simulink model "PX4_Run_Mode_R2017b"  (R2017b)
settings: Solver=FixedStepDiscrete  StartTime=0.0  StopTime=10.0  RelTol=1e-3  EnableMultiTasking=on
InitFcn:
  | run('InitFcn_R2017b_no_csc.m');
values from neighbouring files (symbols this model uses):
  A = Pixhawk_CSC.Parameter( {single([diag([1 1 1]) Ts*diag([1 1 1]); diag([0 0 0]) diag([1 1 1])]),'A'} )    [InitFcn.m]    (also in InitFcn_R2016b.m; InitFcn_R2017b_no_csc.m = single([diag([1 1 1]) Ts*diag([1 1 1]); diag([0 0 0]) diag([)
  app = Pixhawk_CSC.Parameter({single( [0.05; 0.05; 0.05]),'app'} )    [InitFcn.m]    (also in InitFcn_R2016b.m; InitFcn_R2017b_no_csc.m = single( [0.05; 0.05; 0.05]))
  B = Pixhawk_CSC.Parameter( {single([Ts^2/2*diag([1 1 1]); Ts*diag([1 1 1])]),'B'} )    [InitFcn.m]    (also in InitFcn_R2016b.m; InitFcn_R2017b_no_csc.m = single([Ts^2/2*diag([1 1 1]); Ts*diag([1 1 1])]))
  Beta = Pixhawk_CSC.Parameter({single( 0.02),'Beta'} )    [InitFcn.m]    (also in InitFcn_R2016b.m; InitFcn_R2017b_no_csc.m = single( 0.02))
  C = Pixhawk_CSC.Parameter( {single([diag([1 1 1]) 0*diag([1 1 1]); zeros(1,2) 1 zeros(1,3)]),'C'} )    [InitFcn.m]    (also in InitFcn_R2016b.m; InitFcn_R2017b_no_csc.m = single([diag([1 1 1]) 0*diag([1 1 1]); zeros(1,2) 1 zeros(1,)
  C1 = Pixhawk_CSC.Parameter({single( 1.08680),'C1'} )    [InitFcn.m]    (also in InitFcn_R2016b.m; InitFcn_R2017b_no_csc.m = single( 1.08680))
  C10 = Pixhawk_CSC.Parameter({single( 0.0000),'C10'} )    [InitFcn.m]    (also in InitFcn_R2016b.m; InitFcn_R2017b_no_csc.m = single( 0.0000))
  C11 = Pixhawk_CSC.Parameter({single(-0.2300),'C11'} )    [InitFcn.m]    (also in InitFcn_R2016b.m; InitFcn_R2017b_no_csc.m = single(-0.2300))
  C12 = Pixhawk_CSC.Parameter({single( 0.0000),'C12'} )    [InitFcn.m]    (also in InitFcn_R2016b.m; InitFcn_R2017b_no_csc.m = single( 0.0000))
  C13 = Pixhawk_CSC.Parameter({single( 0.8000),'C13'} )    [InitFcn.m]    (also in InitFcn_R2016b.m; InitFcn_R2017b_no_csc.m = single( 0.8000))
  C14 = Pixhawk_CSC.Parameter({single( 0.8000),'C14'} )    [InitFcn.m]    (also in InitFcn_R2016b.m; InitFcn_R2017b_no_csc.m = single( 0.8000))
  C15 = Pixhawk_CSC.Parameter({single( 1.73200),'C15'} )    [InitFcn.m]    (also in InitFcn_R2016b.m; InitFcn_R2017b_no_csc.m = single( 1.73200))
  C16 = Pixhawk_CSC.Parameter({single( 0.1000),'C16'} )    [InitFcn.m]    (also in InitFcn_R2016b.m; InitFcn_R2017b_no_csc.m = single( 0.1000))
  C17 = Pixhawk_CSC.Parameter({single( 0.1000),'C17'} )    [InitFcn.m]    (also in InitFcn_R2016b.m; InitFcn_R2017b_no_csc.m = single( 0.1000))
  C18 = Pixhawk_CSC.Parameter({single( 0.0500),'C18'} )    [InitFcn.m]    (also in InitFcn_R2016b.m; InitFcn_R2017b_no_csc.m = single( 0.0500))
  C19 = Pixhawk_CSC.Parameter({single( 0.6000),'C19'} )    [InitFcn.m]    (also in InitFcn_R2016b.m; InitFcn_R2017b_no_csc.m = single( 0.6000))
  C2 = Pixhawk_CSC.Parameter({single( 1.10468),'C2'} )    [InitFcn.m]    (also in InitFcn_R2016b.m; InitFcn_R2017b_no_csc.m = single( 1.10468))
  C20 = Pixhawk_CSC.Parameter({single( 0.6000),'C20'} )    [InitFcn.m]    (also in InitFcn_R2016b.m; InitFcn_R2017b_no_csc.m = single( 0.6000))
  C21 = Pixhawk_CSC.Parameter({single( 1.04558),'C21'} )    [InitFcn.m]    (also in InitFcn_R2016b.m; InitFcn_R2017b_no_csc.m = single( 1.04558))
  C22 = Pixhawk_CSC.Parameter({single( 0.0000),'C22'} )    [InitFcn.m]    (also in InitFcn_R2016b.m; InitFcn_R2017b_no_csc.m = single( 0.0000))
  C23 = Pixhawk_CSC.Parameter({single( 0.0000),'C23'} )    [InitFcn.m]    (also in InitFcn_R2016b.m; InitFcn_R2017b_no_csc.m = single( 0.0000))
  C24 = Pixhawk_CSC.Parameter({single(-11.0000),'C24'} )    [InitFcn.m]    (also in InitFcn_R2016b.m; InitFcn_R2017b_no_csc.m = single(-11.0000))
  C3 = Pixhawk_CSC.Parameter({single( 1.1980),'C3'} )    [InitFcn.m]    (also in InitFcn_R2016b.m; InitFcn_R2017b_no_csc.m = single( 1.1980))
  C4 = Pixhawk_CSC.Parameter({single( 0.0500),'C4'} )    [InitFcn.m]    (also in InitFcn_R2016b.m; InitFcn_R2017b_no_csc.m = single( 0.0500))
  C5 = Pixhawk_CSC.Parameter({single( 0.0500),'C5'} )    [InitFcn.m]    (also in InitFcn_R2016b.m; InitFcn_R2017b_no_csc.m = single( 0.0500))
  C6 = Pixhawk_CSC.Parameter({single( 0.0500),'C6'} )    [InitFcn.m]    (also in InitFcn_R2016b.m; InitFcn_R2017b_no_csc.m = single( 0.0500))
  C7 = Pixhawk_CSC.Parameter({single( 0.35937),'C7'} )    [InitFcn.m]    (also in InitFcn_R2016b.m; InitFcn_R2017b_no_csc.m = single( 0.35937))
  C8 = Pixhawk_CSC.Parameter({single( 0.36528),'C8'} )    [InitFcn.m]    (also in InitFcn_R2016b.m; InitFcn_R2017b_no_csc.m = single( 0.36528))
  C9 = Pixhawk_CSC.Parameter({single( 0.53311),'C9'} )    [InitFcn.m]    (also in InitFcn_R2016b.m; InitFcn_R2017b_no_csc.m = single( 0.53311))
  C_1 = Pixhawk_CSC.Parameter( {single([diag([1 1 1]) 0*diag([1 1 1])]),'C1'} )    [InitFcn.m]    (also in InitFcn_R2016b.m; InitFcn_R2017b_no_csc.m = single([diag([1 1 1]) 0*diag([1 1 1])]))
  CAL_ACC0_XOFFSET = Pixhawk_CSC.Parameter( {single( 0.122052  ),'CAL_ACC0_XOFFSET'} )    [InitFcn.m]    (also in InitFcn_R2016b.m; InitFcn_R2017b_no_csc.m = single( 0.122052  ))
  CAL_ACC0_XXSCALE = Pixhawk_CSC.Parameter( {single(  1.01218    ),'CAL_ACC0_XXSCALE'} )    [InitFcn.m]    (also in InitFcn_R2016b.m; InitFcn_R2017b_no_csc.m = single(  1.01218    ))
  CAL_ACC0_XYSCALE = Pixhawk_CSC.Parameter( {single( -0.00443301 ),'CAL_ACC0_XYSCALE'} )    [InitFcn.m]    (also in InitFcn_R2016b.m; InitFcn_R2017b_no_csc.m = single( -0.00443301 ))
  CAL_ACC0_XZSCALE = Pixhawk_CSC.Parameter( {single( -0.00505793 ),'CAL_ACC0_XZSCALE'} )    [InitFcn.m]    (also in InitFcn_R2016b.m; InitFcn_R2017b_no_csc.m = single( -0.00505793 ))
  CAL_ACC0_YOFFSET = Pixhawk_CSC.Parameter( {single( 0.00281205),'CAL_ACC0_YOFFSET'} )    [InitFcn.m]    (also in InitFcn_R2016b.m; InitFcn_R2017b_no_csc.m = single( 0.00281205))
  CAL_ACC0_YXSCALE = Pixhawk_CSC.Parameter( {single( -0.00443301 ),'CAL_ACC0_YXSCALE'} )    [InitFcn.m]    (also in InitFcn_R2016b.m; InitFcn_R2017b_no_csc.m = single( -0.00443301 ))
  CAL_ACC0_YYSCALE = Pixhawk_CSC.Parameter( {single(  1.00234    ),'CAL_ACC0_YYSCALE'} )    [InitFcn.m]    (also in InitFcn_R2016b.m; InitFcn_R2017b_no_csc.m = single(  1.00234    ))
  CAL_ACC0_YZSCALE = Pixhawk_CSC.Parameter( {single(  0.0160883  ),'CAL_ACC0_YZSCALE'} )    [InitFcn.m]    (also in InitFcn_R2016b.m; InitFcn_R2017b_no_csc.m = single(  0.0160883  ))
  CAL_ACC0_ZOFFSET = Pixhawk_CSC.Parameter( {single(-0.0298121 ),'CAL_ACC0_ZOFFSET'} )    [InitFcn.m]    (also in InitFcn_R2016b.m; InitFcn_R2017b_no_csc.m = single(-0.0298121 ))
  CAL_ACC0_ZXSCALE = Pixhawk_CSC.Parameter( {single( -0.00505793 ),'CAL_ACC0_ZXSCALE'} )    [InitFcn.m]    (also in InitFcn_R2016b.m; InitFcn_R2017b_no_csc.m = single( -0.00505793 ))
  CAL_ACC0_ZYSCALE = Pixhawk_CSC.Parameter( {single(  0.0160883  ),'CAL_ACC0_ZYSCALE'} )    [InitFcn.m]    (also in InitFcn_R2016b.m; InitFcn_R2017b_no_csc.m = single(  0.0160883  ))
  CAL_ACC0_ZZSCALE = Pixhawk_CSC.Parameter( {single(  0.983604   ),'CAL_ACC0_ZZSCALE'} )    [InitFcn.m]    (also in InitFcn_R2016b.m; InitFcn_R2017b_no_csc.m = single(  0.983604   ))
  CAL_BAR_OFFSET = Pixhawk_CSC.Parameter( {single( -20.8468),'CAL_BAR_OFFSET'} )    [InitFcn.m]    (also in InitFcn_R2016b.m; InitFcn_R2017b_no_csc.m = single( -20.8468))
  CAL_BAR_SCALE = Pixhawk_CSC.Parameter( {single(   1.0632),'CAL_BAR_SCALE'} )    [InitFcn.m]    (also in InitFcn_R2016b.m; InitFcn_R2017b_no_csc.m = single(   1.0632))
  CAL_BAT0_XOFFSET = Pixhawk_CSC.Parameter( {single( 0.0000),'CAL_BAT0_XOFFSET'} )    [InitFcn.m]    (also in InitFcn_R2016b.m; InitFcn_R2017b_no_csc.m = single( 0.0000))
  CAL_BAT0_XXSCALE = Pixhawk_CSC.Parameter( {single(  1.0000),'CAL_BAT0_XXSCALE'} )    [InitFcn.m]    (also in InitFcn_R2016b.m; InitFcn_R2017b_no_csc.m = single(  1.0000))
  CAL_BAT0_XYSCALE = Pixhawk_CSC.Parameter( {single(  0.0000),'CAL_BAT0_XYSCALE'} )    [InitFcn.m]    (also in InitFcn_R2016b.m; InitFcn_R2017b_no_csc.m = single(  0.0000))
  CAL_BAT0_XZSCALE = Pixhawk_CSC.Parameter( {single(  0.0000),'CAL_BAT0_XZSCALE'} )    [InitFcn.m]    (also in InitFcn_R2016b.m; InitFcn_R2017b_no_csc.m = single(  0.0000))
  CAL_BAT0_YOFFSET = Pixhawk_CSC.Parameter( {single( 0.0000),'CAL_BAT0_YOFFSET'} )    [InitFcn.m]    (also in InitFcn_R2016b.m; InitFcn_R2017b_no_csc.m = single( 0.0000))
  CAL_BAT0_YXSCALE = Pixhawk_CSC.Parameter( {single(  0.0000),'CAL_BAT0_YXSCALE'} )    [InitFcn.m]    (also in InitFcn_R2016b.m; InitFcn_R2017b_no_csc.m = single(  0.0000))
  CAL_BAT0_YYSCALE = Pixhawk_CSC.Parameter( {single(  1.0000),'CAL_BAT0_YYSCALE'} )    [InitFcn.m]    (also in InitFcn_R2016b.m; InitFcn_R2017b_no_csc.m = single(  1.0000))
  CAL_BAT0_YZSCALE = Pixhawk_CSC.Parameter( {single(  0.0000),'CAL_BAT0_YZSCALE'} )    [InitFcn.m]    (also in InitFcn_R2016b.m; InitFcn_R2017b_no_csc.m = single(  0.0000))
  CAL_BAT0_ZOFFSET = Pixhawk_CSC.Parameter( {single( 0.0000),'CAL_BAT0_ZOFFSET'} )    [InitFcn.m]    (also in InitFcn_R2016b.m; InitFcn_R2017b_no_csc.m = single( 0.0000))
  CAL_BAT0_ZXSCALE = Pixhawk_CSC.Parameter( {single(  0.0000),'CAL_BAT0_ZXSCALE'} )    [InitFcn.m]    (also in InitFcn_R2016b.m; InitFcn_R2017b_no_csc.m = single(  0.0000))
  CAL_BAT0_ZYSCALE = Pixhawk_CSC.Parameter( {single(  0.0000),'CAL_BAT0_ZYSCALE'} )    [InitFcn.m]    (also in InitFcn_R2016b.m; InitFcn_R2017b_no_csc.m = single(  0.0000))
  CAL_BAT0_ZZSCALE = Pixhawk_CSC.Parameter( {single(  1.0000),'CAL_BAT0_ZZSCALE'} )    [InitFcn.m]    (also in InitFcn_R2016b.m; InitFcn_R2017b_no_csc.m = single(  1.0000))
  CAL_GPS0_XOFFSET = Pixhawk_CSC.Parameter( {single( 0.0000),'CAL_GPS0_XOFFSET'} )    [InitFcn.m]    (also in InitFcn_R2016b.m; InitFcn_R2017b_no_csc.m = single( 0.0000))
  CAL_GPS0_XXSCALE = Pixhawk_CSC.Parameter( {single(  0.0100),'CAL_GPS0_XXSCALE'} )    [InitFcn.m]    (also in InitFcn_R2016b.m; InitFcn_R2017b_no_csc.m = single(  0.0100))
  CAL_GPS0_XYSCALE = Pixhawk_CSC.Parameter( {single(  0.0000),'CAL_GPS0_XYSCALE'} )    [InitFcn.m]    (also in InitFcn_R2016b.m; InitFcn_R2017b_no_csc.m = single(  0.0000))
  CAL_GPS0_XZSCALE = Pixhawk_CSC.Parameter( {single(  0.0000),'CAL_GPS0_XZSCALE'} )    [InitFcn.m]    (also in InitFcn_R2016b.m; InitFcn_R2017b_no_csc.m = single(  0.0000))
  CAL_GPS0_YOFFSET = Pixhawk_CSC.Parameter( {single( 0.0000),'CAL_GPS0_YOFFSET'} )    [InitFcn.m]    (also in InitFcn_R2016b.m; InitFcn_R2017b_no_csc.m = single( 0.0000))
  CAL_GPS0_YXSCALE = Pixhawk_CSC.Parameter( {single(  0.0000),'CAL_GPS0_YXSCALE'} )    [InitFcn.m]    (also in InitFcn_R2016b.m; InitFcn_R2017b_no_csc.m = single(  0.0000))
  CAL_GPS0_YYSCALE = Pixhawk_CSC.Parameter( {single(  0.0100),'CAL_GPS0_YYSCALE'} )    [InitFcn.m]    (also in InitFcn_R2016b.m; InitFcn_R2017b_no_csc.m = single(  0.0100))
  CAL_GPS0_YZSCALE = Pixhawk_CSC.Parameter( {single(  0.0000),'CAL_GPS0_YZSCALE'} )    [InitFcn.m]    (also in InitFcn_R2016b.m; InitFcn_R2017b_no_csc.m = single(  0.0000))
  CAL_GPS0_ZOFFSET = Pixhawk_CSC.Parameter( {single( 0.0000),'CAL_GPS0_ZOFFSET'} )    [InitFcn.m]    (also in InitFcn_R2016b.m; InitFcn_R2017b_no_csc.m = single( 0.0000))
  CAL_GPS0_ZXSCALE = Pixhawk_CSC.Parameter( {single(  0.0000),'CAL_GPS0_ZXSCALE'} )    [InitFcn.m]    (also in InitFcn_R2016b.m; InitFcn_R2017b_no_csc.m = single(  0.0000))
  CAL_GPS0_ZYSCALE = Pixhawk_CSC.Parameter( {single(  0.0000),'CAL_GPS0_ZYSCALE'} )    [InitFcn.m]    (also in InitFcn_R2016b.m; InitFcn_R2017b_no_csc.m = single(  0.0000))
  CAL_GPS0_ZZSCALE = Pixhawk_CSC.Parameter( {single( -0.0010),'CAL_GPS0_ZZSCALE'} )    [InitFcn.m]    (also in InitFcn_R2016b.m; InitFcn_R2017b_no_csc.m = single( -0.0010))
  CAL_GYRO0_XXSCALE = Pixhawk_CSC.Parameter( {single(0.992736),'CAL_GYRO0_XXSCALE'} )    [InitFcn.m]    (also in InitFcn_R2016b.m; InitFcn_R2017b_no_csc.m = single(0.992736))
  CAL_GYRO0_XYSCALE = Pixhawk_CSC.Parameter( {single(0.0000),'CAL_GYRO0_XYSCALE'} )    [InitFcn.m]    (also in InitFcn_R2016b.m; InitFcn_R2017b_no_csc.m = single(0.0000))
  CAL_GYRO0_XZSCALE = Pixhawk_CSC.Parameter( {single(0.0000),'CAL_GYRO0_XZSCALE'} )    [InitFcn.m]    (also in InitFcn_R2016b.m; InitFcn_R2017b_no_csc.m = single(0.0000))
  CAL_GYRO0_YXSCALE = Pixhawk_CSC.Parameter( {single(0.0000),'CAL_GYRO0_YXSCALE'} )    [InitFcn.m]    (also in InitFcn_R2016b.m; InitFcn_R2017b_no_csc.m = single(0.0000))
  CAL_GYRO0_YYSCALE = Pixhawk_CSC.Parameter( {single(1.01609),'CAL_GYRO0_YYSCALE'} )    [InitFcn.m]    (also in InitFcn_R2016b.m; InitFcn_R2017b_no_csc.m = single(1.01609))
  CAL_GYRO0_YZSCALE = Pixhawk_CSC.Parameter( {single(0.0000),'CAL_GYRO0_YZSCALE'} )    [InitFcn.m]    (also in InitFcn_R2016b.m; InitFcn_R2017b_no_csc.m = single(0.0000))
  CAL_GYRO0_ZXSCALE = Pixhawk_CSC.Parameter( {single(0.0000),'CAL_GYRO0_ZXSCALE'} )    [InitFcn.m]    (also in InitFcn_R2016b.m; InitFcn_R2017b_no_csc.m = single(0.0000))
  CAL_GYRO0_ZYSCALE = Pixhawk_CSC.Parameter( {single(0.0000),'CAL_GYRO0_ZYSCALE'} )    [InitFcn.m]    (also in InitFcn_R2016b.m; InitFcn_R2017b_no_csc.m = single(0.0000))
  CAL_GYRO0_ZZSCALE = Pixhawk_CSC.Parameter( {single(1.03003),'CAL_GYRO0_ZZSCALE'} )    [InitFcn.m]    (also in InitFcn_R2016b.m; InitFcn_R2017b_no_csc.m = single(1.03003))
  CAL_MAG0_XCURCOR = Pixhawk_CSC.Parameter( {single( 0.0017     ),'CAL_MAG0_XCURCOR'} )    [InitFcn.m]    (also in InitFcn_R2016b.m; InitFcn_R2017b_no_csc.m = single( 0.0017     ))
  CAL_MAG0_XOFFSET = Pixhawk_CSC.Parameter( {single( 0.0446372  ),'CAL_MAG0_XOFFSET'} )    [InitFcn.m]    (also in InitFcn_R2016b.m; InitFcn_R2017b_no_csc.m = single( 0.0446372  ))
  CAL_MAG0_XXSCALE = Pixhawk_CSC.Parameter( {single(  1.01563   ),'CAL_MAG0_XXSCALE'} )    [InitFcn.m]    (also in InitFcn_R2016b.m; InitFcn_R2017b_no_csc.m = single(  1.01563   ))
  CAL_MAG0_XYSCALE = Pixhawk_CSC.Parameter( {single( -0.0612061 ),'CAL_MAG0_XYSCALE'} )    [InitFcn.m]    (also in InitFcn_R2016b.m; InitFcn_R2017b_no_csc.m = single( -0.0612061 ))
  CAL_MAG0_XZSCALE = Pixhawk_CSC.Parameter( {single( -0.011532  ),'CAL_MAG0_XZSCALE'} )    [InitFcn.m]    (also in InitFcn_R2016b.m; InitFcn_R2017b_no_csc.m = single( -0.011532  ))
  CAL_MAG0_YCURCOR = Pixhawk_CSC.Parameter( {single(-0.0075     ),'CAL_MAG0_YCURCOR'} )    [InitFcn.m]    (also in InitFcn_R2016b.m; InitFcn_R2017b_no_csc.m = single(-0.0075     ))
  CAL_MAG0_YOFFSET = Pixhawk_CSC.Parameter( {single( 0.0700776  ),'CAL_MAG0_YOFFSET'} )    [InitFcn.m]    (also in InitFcn_R2016b.m; InitFcn_R2017b_no_csc.m = single( 0.0700776  ))
  CAL_MAG0_YXSCALE = Pixhawk_CSC.Parameter( {single( -0.0612061 ),'CAL_MAG0_YXSCALE'} )    [InitFcn.m]    (also in InitFcn_R2016b.m; InitFcn_R2017b_no_csc.m = single( -0.0612061 ))
  CAL_MAG0_YYSCALE = Pixhawk_CSC.Parameter( {single(  1.00593   ),'CAL_MAG0_YYSCALE'} )    [InitFcn.m]    (also in InitFcn_R2016b.m; InitFcn_R2017b_no_csc.m = single(  1.00593   ))
  CAL_MAG0_YZSCALE = Pixhawk_CSC.Parameter( {single(  0.0144582 ),'CAL_MAG0_YZSCALE'} )    [InitFcn.m]    (also in InitFcn_R2016b.m; InitFcn_R2017b_no_csc.m = single(  0.0144582 ))
  CAL_MAG0_ZCURCOR = Pixhawk_CSC.Parameter( {single(-0.0080     ),'CAL_MAG0_ZCURCOR'} )    [InitFcn.m]    (also in InitFcn_R2016b.m; InitFcn_R2017b_no_csc.m = single(-0.0080     ))
  CAL_MAG0_ZOFFSET = Pixhawk_CSC.Parameter( {single( 0.00201742 ),'CAL_MAG0_ZOFFSET'} )    [InitFcn.m]    (also in InitFcn_R2016b.m; InitFcn_R2017b_no_csc.m = single( 0.00201742 ))
  CAL_MAG0_ZXSCALE = Pixhawk_CSC.Parameter( {single( -0.011532  ),'CAL_MAG0_ZXSCALE'} )    [InitFcn.m]    (also in InitFcn_R2016b.m; InitFcn_R2017b_no_csc.m = single( -0.011532  ))
  CAL_MAG0_ZYSCALE = Pixhawk_CSC.Parameter( {single(  0.0144582 ),'CAL_MAG0_ZYSCALE'} )    [InitFcn.m]    (also in InitFcn_R2016b.m; InitFcn_R2017b_no_csc.m = single(  0.0144582 ))
  CAL_MAG0_ZZSCALE = Pixhawk_CSC.Parameter( {single(  0.986813  ),'CAL_MAG0_ZZSCALE'} )    [InitFcn.m]    (also in InitFcn_R2016b.m; InitFcn_R2017b_no_csc.m = single(  0.986813  ))
  CAL_SONAR_OFFSET = Pixhawk_CSC.Parameter( {single( -6.8730),'CAL_SONAR_OFFSET'} )    [InitFcn.m]    (also in InitFcn_R2016b.m; InitFcn_R2017b_no_csc.m = single( -6.8730))
  CAL_SONAR_SCALE = Pixhawk_CSC.Parameter( {single(-438.1875),'CAL_SONAR_SCALE'} )    [InitFcn.m]    (also in InitFcn_R2016b.m; InitFcn_R2017b_no_csc.m = single(-438.1875))
  COM_RATE = double(10)    [InitFcn.m]    (also in InitFcn_R2016b.m; InitFcn_R2017b_no_csc.m)
  D = Pixhawk_CSC.Parameter( {single(zeros(size(C.Value,1), size(B.Value,2))),'D'} )    [InitFcn.m]    (also in InitFcn_R2016b.m; InitFcn_R2017b_no_csc.m = single(zeros(size(C,1), size(B,2))))
  Dip0 = Pixhawk_CSC.Parameter({single( 1.2),'Dip0'} )    [InitFcn.m]    (also in InitFcn_R2016b.m; InitFcn_R2017b_no_csc.m = single( 1.2))
  I = Pixhawk_CSC.Parameter( {single(eye(size(Q.Value))),'I'} )    [InitFcn.m]    (also in InitFcn_R2016b.m; InitFcn_R2017b_no_csc.m = single(eye(size(Q))))
  Jxx = Pixhawk_CSC.Parameter( {single(J(1,1)),'Jxx'} )    [InitFcn.m]    (also in InitFcn_R2016b.m; InitFcn_R2017b_no_csc.m = single(J(1,1)))
  Jyy = Pixhawk_CSC.Parameter( {single(J(2,2)),'Jyy'} )    [InitFcn.m]    (also in InitFcn_R2016b.m; InitFcn_R2017b_no_csc.m = single(J(2,2)))
  Jzz = Pixhawk_CSC.Parameter( {single(J(3,3)),'Jzz'} )    [InitFcn.m]    (also in InitFcn_R2016b.m; InitFcn_R2017b_no_csc.m = single(J(3,3)))
  Kapp = Pixhawk_CSC.Parameter({single( 1.2),'Kapp'} )    [InitFcn.m]    (also in InitFcn_R2016b.m; InitFcn_R2017b_no_csc.m = single( 1.2))
  Kx = Pixhawk_CSC.Parameter({single( Kx),'Kx'} )    [InitFcn.m]    (also in InitFcn_R2016b.m = Pixhawk_CSC.Parameter({single( [0.60 0.9]),'Kx'} ); InitFcn_R2017b_no_csc.m = single( [0.60 0.9]))
  Ky = Pixhawk_CSC.Parameter({single( Ky),'Ky'} )    [InitFcn.m]    (also in InitFcn_R2016b.m = Pixhawk_CSC.Parameter({single( [0.4 0.9]),'Ky'} ); InitFcn_R2017b_no_csc.m = single( [0.4 0.9]))
  LPF_REF_DEN = Pixhawk_CSC.Parameter( {single([1.0000 -0.8187]),'LPF_REF_DEN'} )    [InitFcn.m]    (also in InitFcn_R2016b.m; InitFcn_R2017b_no_csc.m = single([1.0000 -0.8187]))
  LPF_REF_NUM = Pixhawk_CSC.Parameter( {single([0.0000  0.1813]),'LPF_REF_NUM'} )    [InitFcn.m]    (also in InitFcn_R2016b.m; InitFcn_R2017b_no_csc.m = single([0.0000  0.1813]))
  m0 = Pixhawk_CSC.Parameter({single( 0.452857),'m0'} )    [InitFcn.m]    (also in InitFcn_R2016b.m; InitFcn_R2017b_no_csc.m = single( 0.452857))
  mn = [0.01; 0.01; 0.01; 0.01]    [InitFcn.m]    (also in InitFcn_R2016b.m; InitFcn_R2017b_no_csc.m)
  MOV_AVG_WINDOW = Pixhawk_CSC.Parameter( {single(100),'MOV_AVG_WINDOW'} )    [InitFcn.m]    (also in InitFcn_R2016b.m; InitFcn_R2017b_no_csc.m = single(100))
  Ox0 = Pixhawk_CSC.Parameter({single(O_x0),'Ox0'} )    [InitFcn.m]    (also in InitFcn_R2016b.m; InitFcn_R2017b_no_csc.m = single(O_x0))
  Oxa = Pixhawk_CSC.Parameter({single(O_x.a),'Oxa'} )    [InitFcn.m]    (also in InitFcn_R2016b.m; InitFcn_R2017b_no_csc.m = single(O_x.a))
  Oxb = Pixhawk_CSC.Parameter({single(O_x.b),'Oxb'} )    [InitFcn.m]    (also in InitFcn_R2016b.m; InitFcn_R2017b_no_csc.m = single(O_x.b))
  Oxc = Pixhawk_CSC.Parameter({single(O_x.c),'Oxc'} )    [InitFcn.m]    (also in InitFcn_R2016b.m; InitFcn_R2017b_no_csc.m = single(O_x.c))
  Oxd = Pixhawk_CSC.Parameter({single(O_x.d),'Oxd'} )    [InitFcn.m]    (also in InitFcn_R2016b.m; InitFcn_R2017b_no_csc.m = single(O_x.d))
  Oy0 = Pixhawk_CSC.Parameter({single(O_y0),'Oy0'} )    [InitFcn.m]    (also in InitFcn_R2016b.m; InitFcn_R2017b_no_csc.m = single(O_y0))
  Oya = Pixhawk_CSC.Parameter({single(O_y.a),'Oya'} )    [InitFcn.m]    (also in InitFcn_R2016b.m; InitFcn_R2017b_no_csc.m = single(O_y.a))
  Oyb = Pixhawk_CSC.Parameter({single(O_y.b),'Oyb'} )    [InitFcn.m]    (also in InitFcn_R2016b.m; InitFcn_R2017b_no_csc.m = single(O_y.b))
  Oyc = Pixhawk_CSC.Parameter({single(O_y.c),'Oyc'} )    [InitFcn.m]    (also in InitFcn_R2016b.m; InitFcn_R2017b_no_csc.m = single(O_y.c))
  Oyd = Pixhawk_CSC.Parameter({single(O_y.d),'Oyd'} )    [InitFcn.m]    (also in InitFcn_R2016b.m; InitFcn_R2017b_no_csc.m = single(O_y.d))
  Oz0 = Pixhawk_CSC.Parameter({single(O_z0),'Oz0'} )    [InitFcn.m]    (also in InitFcn_R2016b.m; InitFcn_R2017b_no_csc.m = single(O_z0))
  ... (+53 more)
undefined symbols (not defined in the file or in its folder): AccX, AccY, AccZ, Altitude, ax, ay, az, Current, FILTER_N, GPS_TS, GyroX, GyroY, GyroZ, Latitude, Longitude, M1_PWM, M2_PWM, M3_PWM, M4_PWM, MagX, MagY, MagZ, mAH, MOTOR, phi, Position_TS, psi, PX4_TUNE_ENUM, RGBLED_COLOR_ENUM, RGBLED_MODE_ENUM, S_AccX, S_AccY, S_AccZ, S_Altitude, S_Baro, S_Current, S_GyroX, S_GyroY, S_GyroZ, S_Latitude, S_Longitude, S_MagX, S_MagY, S_MagZ, S_mAH, S_N_Sat, S_Voltage, T_PITCH, T_ROLL, T_THROTTLE, theta, v, Voltage, w, wx, wxd, wy, wyd, wz ... (+4)
libraries: simulink x31, pixhawk_slib_sensors_actuators x7, pixhawk_slib_ADC_serial x5, pixhawk_slib_misc_utils x3, etargetslib x2
(part 6 of 7)

== system PX4_Run_Mode_R2017b/SENSOR_FILTER/Fixed Bias removal and scaling/Parameter Bus Creation/Kalman Filter/C matrix ==
  C matrix In : Inport
  Bus Creator : BusCreator  Inputs=24
  Data Type Conversion : DataTypeConversion  OutDataTypeStr=single
  Demux : Demux  Outputs=24
  C matrix Out : Outport
  wires:
  C matrix In/1 -> Data Type Conversion/1
  Bus Creator/1 -> C matrix Out/1  "C matrix"
  Demux/8 -> Bus Creator/8  "C42"
  Demux/10 -> Bus Creator/10  "C23"
  Demux/5 -> Bus Creator/5  "C12"
  Demux/13 -> Bus Creator/13  "C14"
  Demux/9 -> Bus Creator/9  "C13"
  Demux/18 -> Bus Creator/18  "C25"
  Demux/6 -> Bus Creator/6  "C22"
  Demux/12 -> Bus Creator/12  "C43"
  Demux/4 -> Bus Creator/4  "C41"
  Demux/7 -> Bus Creator/7  "C32"
  Demux/17 -> Bus Creator/17  "C15"
  Demux/11 -> Bus Creator/11  "C33"
  Demux/15 -> Bus Creator/15  "C34"
  Demux/3 -> Bus Creator/3  "C31"
  Demux/14 -> Bus Creator/14  "C24"
  Demux/16 -> Bus Creator/16  "C44"
  Demux/2 -> Bus Creator/2  "C21"
  Demux/1 -> Bus Creator/1  "C11"
  Data Type Conversion/1 -> Demux/1
  Demux/22 -> Bus Creator/22  "C26"
  Demux/23 -> Bus Creator/23  "C36"
  Demux/20 -> Bus Creator/20  "C45"
  Demux/19 -> Bus Creator/19  "C35"
  Demux/21 -> Bus Creator/21  "C16"
  Demux/24 -> Bus Creator/24  "C46"

== system PX4_Run_Mode_R2017b/SENSOR_FILTER/Fixed Bias removal and scaling/Parameter Bus Creation/Kalman Filter/D matrix ==
  D matrix In : Inport
  Bus Creator : BusCreator  Inputs=12
  Data Type Conversion : DataTypeConversion  OutDataTypeStr=single
  Demux : Demux  Outputs=12
  D matrix Out : Outport
  wires:
  D matrix In/1 -> Data Type Conversion/1
  Bus Creator/1 -> D matrix Out/1  "D matrix"
  Demux/8 -> Bus Creator/8  "D42"
  Demux/5 -> Bus Creator/5  "D12"
  Demux/9 -> Bus Creator/9  "D13"
  Demux/6 -> Bus Creator/6  "D22"
  Demux/4 -> Bus Creator/4  "D41"
  Demux/7 -> Bus Creator/7  "D32"
  Demux/3 -> Bus Creator/3  "D31"
  Demux/2 -> Bus Creator/2  "D21"
  Demux/1 -> Bus Creator/1  "D11"
  Data Type Conversion/1 -> Demux/1
  Demux/10 -> Bus Creator/10  "D23"
  Demux/11 -> Bus Creator/11  "D33"
  Demux/12 -> Bus Creator/12  "D43"

== system PX4_Run_Mode_R2017b/SENSOR_FILTER/Fixed Bias removal and scaling/Parameter Bus Creation/Kalman Filter/Q matrix ==
  Q matrix In : Inport
  Bus Creator : BusCreator  Inputs=36
  Data Type Conversion : DataTypeConversion  OutDataTypeStr=single
  Demux : Demux  Outputs=36
  Q matrix Out : Outport
  wires:
  Q matrix In/1 -> Data Type Conversion/1
  Bus Creator/1 -> Q matrix Out/1  "Q matrix"
  Demux/8 -> Bus Creator/8  "Q22"
  Demux/10 -> Bus Creator/10  "Q42"
  Demux/19 -> Bus Creator/19  "Q14"
  Demux/5 -> Bus Creator/5  "Q51"
  Demux/13 -> Bus Creator/13  "Q13"
  Demux/20 -> Bus Creator/20  "Q24"
  Demux/9 -> Bus Creator/9  "Q32"
  Demux/18 -> Bus Creator/18  "Q63"
  Demux/6 -> Bus Creator/6  "Q61"
  Demux/12 -> Bus Creator/12  "Q62"
  Demux/4 -> Bus Creator/4  "Q41"
  Demux/7 -> Bus Creator/7  "Q12"
  Demux/17 -> Bus Creator/17  "Q53"
  Demux/11 -> Bus Creator/11  "Q52"
  Demux/15 -> Bus Creator/15  "Q33"
  Demux/3 -> Bus Creator/3  "Q31"
  Demux/21 -> Bus Creator/21  "Q34"
  Demux/14 -> Bus Creator/14  "Q23"
  Demux/16 -> Bus Creator/16  "Q43"
  Demux/34 -> Bus Creator/34  "Q46"
  Demux/28 -> Bus Creator/28  "Q45"
  Demux/30 -> Bus Creator/30  "Q65"
  Demux/27 -> Bus Creator/27  "Q35"
  Demux/29 -> Bus Creator/29  "Q55"
  Demux/31 -> Bus Creator/31  "Q16"
  Demux/32 -> Bus Creator/32  "Q26"
  Demux/22 -> Bus Creator/22  "Q44"
  Demux/24 -> Bus Creator/24  "Q64"
  Demux/33 -> Bus Creator/33  "Q36"
  Demux/23 -> Bus Creator/23  "Q54"
  Demux/36 -> Bus Creator/36  "Q66"
  Demux/25 -> Bus Creator/25  "Q15"
  Demux/26 -> Bus Creator/26  "Q25"
  Demux/35 -> Bus Creator/35  "Q56"
  Demux/2 -> Bus Creator/2  "Q21"
  Demux/1 -> Bus Creator/1  "Q11"
  Data Type Conversion/1 -> Demux/1

== system PX4_Run_Mode_R2017b/SENSOR_FILTER/Fixed Bias removal and scaling/Parameter Bus Creation/Kalman Filter/R matrix ==
  R matrix In : Inport
  Bus Creator : BusCreator  Inputs=16
  Data Type Conversion : DataTypeConversion  OutDataTypeStr=single
  Demux : Demux  Outputs=16
  R matrix Out : Outport
  wires:
  R matrix In/1 -> Data Type Conversion/1
  Bus Creator/1 -> R matrix Out/1  "R matrix"
  Demux/8 -> Bus Creator/8  "R42"
  Demux/5 -> Bus Creator/5  "R12"
  Demux/9 -> Bus Creator/9  "R13"
  Demux/6 -> Bus Creator/6  "R22"
  Demux/4 -> Bus Creator/4  "R41"
  Demux/7 -> Bus Creator/7  "R32"
  Demux/3 -> Bus Creator/3  "R31"
  Demux/2 -> Bus Creator/2  "R21"
  Demux/1 -> Bus Creator/1  "R11"
  Data Type Conversion/1 -> Demux/1
  Demux/10 -> Bus Creator/10  "R23"
  Demux/11 -> Bus Creator/11  "R33"
  Demux/12 -> Bus Creator/12  "R43"
  Demux/13 -> Bus Creator/13  "R14"
  Demux/14 -> Bus Creator/14  "R24"
  Demux/15 -> Bus Creator/15  "R34"
  Demux/16 -> Bus Creator/16  "R44"

== matlab function PX4_Run_Mode_R2017b/MOTOR_MIXING & MODE_SELECTOR/Motor Configuration ==
  data: M1_IN input; M2_IN input; M3_IN input; M4_IN input; THRUST input; CONFIG_CMD_IN input; CONFIG_M1 input; CONFIG_M2 input; M1_OUT output; M2_OUT output; M3_OUT output; M4_OUT output; Motor output; CONFIG_M3 input; CONFIG_M4 input
function [M1_OUT, M2_OUT, M3_OUT, M4_OUT, Motor] = Configuration_Check(M1_IN, M2_IN, M3_IN, M4_IN, THRUST, CONFIG_CMD_IN, CONFIG_M1, CONFIG_M2, CONFIG_M3, CONFIG_M4)

%% Set outputs to 0
M1_OUT = uint16(0);
M2_OUT = uint16(0);
M3_OUT = uint16(0);
M4_OUT = uint16(0);
Motor  = uint16(0);
Thrust = uint16(0);

%% IF drone is put into configuration mode:
%         SC
%       H   L
% SD H  FL  BL
%    L  FR  BR
% Where H/L = High/Low bit
%       F/B = Front/Back motors
%       R/L = Right/Left motors
%% Else, normal procedure will be passed through
% If configuration mode is entered, start connecting motors seperatly to
% the thrust

% Test which actuation scheme is entered
if(CONFIG_CMD_IN >= 1)
    if(CONFIG_M1)
        % Test motor 1 Front Right CCW
        Motor = uint16(1);
    elseif(CONFIG_M2)
        % Test motor 2 Back Right CW
        Motor = uint16(2);
    elseif(CONFIG_M3)
        % Test motor 3 Back Left CCW
        Motor = uint16(3);
    elseif(CONFIG_M4)
        % Test motor 4 FRONT Left CW
        Motor = uint16(4);
    else
        % Error, no mode selected
        Motor = uint16(0);
    end
else
    Motor = uint16(5);
end

% Copying
Thrust = THRUST;
% Steps of 100 pwm 
% if(Motor ~= 5 || Motor ~= 0)
%     Thrust = round(THRUST/100)*100;
% end

%% Switch case, where case 0 is used for unknown state
switch Motor
    case uint16(0)             % No motor actuated
        M1_OUT = uint16(1000);
        M2_OUT = uint16(1000);
        M3_OUT = uint16(1000);
        M4_OUT = uint16(1000);
        
    case uint16(1)             % Motor 1 actuated
%         M1_OUT = uint16(round(M1_IN/100)*100);
        M1_OUT = uint16(Thrust);
        M2_OUT = uint16(1000);
        M3_OUT = uint16(1000);
        M4_OUT = uint16(1000);
        
    case uint16(2)             % Motor 2 actuated
        M1_OUT = uint16(1000);
%         M2_OUT = uint16(round(M2_IN/100)*100);
        M2_OUT = uint16(Thrust);
        M3_OUT = uint16(1000);
        M4_OUT = uint16(1000);
        
    case uint16(3)             % Motor 3 actuated
        M1_OUT = uint16(1000);
        M2_OUT = uint16(1000);
%         M3_OUT = uint16(round(M3_IN/100)*100);
        M3_OUT = uint16(Thrust);
        M4_OUT = uint16(1000);
        
    case uint16(4)             % Motor 4 actuated
        M1_OUT = uint16(1000);
        M2_OUT = uint16(1000);
        M3_OUT = uint16(1000);
%         M4_OUT = uint16(round(M4_IN/100)*100);
        M4_OUT = uint16(Thrust);
        
    case uint16(5)             % Actuate all motors
        M1_OUT = uint16(M1_IN);
        M2_OUT = uint16(M2_IN);
        M3_OUT = uint16(M3_IN);
        M4_OUT = uint16(M4_IN);
end

== matlab function PX4_Run_Mode_R2017b/SENSOR_FILTER/Fixed Bias removal and scaling/Barometer Calibration/MATLAB Function ==
  data: BAR_In input; BAR_Out output; CAL_BAR_SCALE parameter; CAL_BAR_OFFSET parameter
function BAR_Out = Barometer_Correction(BAR_In, CAL_BAR_SCALE, CAL_BAR_OFFSET)

BAR_Out = single(1/CAL_BAR_SCALE*(BAR_In - CAL_BAR_OFFSET));

== matlab function PX4_Run_Mode_R2017b/SENSOR_FILTER/Bias Removal State/MATLAB Function3 ==
  data: STATE_IN input; RESET input; STATE_OUT output; CONFIG_CMD input; MOV_AVG_WINDOW parameter; BIAS_STATE output
function [STATE_OUT, BIAS_STATE] = StateBias(STATE_IN, RESET, CONFIG_CMD, MOV_AVG_WINDOW)

%% Initiate BIAS Memory
persistent BIAS;
if(isempty(BIAS) || RESET)
    BIAS = single([0; 0; 0;... 
                   0; 0; 0;... 
                   0; 0; 0;... 
                   0; 0; 0;... 
                   0; 0; 0;... 
                   0; 0; 0]);
end

BIAS_STATE = single([0; 0; 0;... 
                     0; 0; 0;... 
                     0; 0; 0;... 
                     0; 0; 0;... 
                     0; 0; 0;... 
                     0; 0; 0]);

%% If Pre-Armed, average input
if(CONFIG_CMD)
    BIAS = BIAS + STATE_IN/MOV_AVG_WINDOW;
end

%% Remove BIAS from input
% BIAS([4 5 6]) = [0 0 0];
STATE_OUT = STATE_IN - BIAS;
BIAS_STATE = BIAS;

== matlab function PX4_Run_Mode_R2017b/SENSOR_FILTER/StateEstimatesInitialConditions/State Estimater Initial Conditions ==
  data: Xhat output
function Xhat = StateEstimatorInitialConditions

Xhat = single([0; 0; 0;...     % Positions
               0; 0; 0;...     % Angles
               0; 0; 0;...     % Velocities
               0; 0; 0;...     % Angular velocities
               0; 0; 0;...     % Accelerations
               0; 0; 0]);      % Angular accelerations

== matlab function PX4_Run_Mode_R2017b/RC_FILTER/PWM2THRUST ==
  data: THROTTLE_CONTROL_INPUT input; THROTTLE_CONTROL_OUTPUT output; PWM_a parameter; PWM_b parameter; PWM_c parameter; PWM_d parameter
function THROTTLE_CONTROL_OUTPUT = PWM2THRUST(THROTTLE_CONTROL_INPUT, PWM_a, PWM_b, PWM_c, PWM_d)

a = single(PWM_a);
b = single(PWM_b);
c = single(PWM_c);
d = single(PWM_d);

PWM = single(THROTTLE_CONTROL_INPUT);
THROTTLE_CONTROL_OUTPUT = single(0);

%% Convert PWM to Thrust
THROTTLE_CONTROL_OUTPUT = -4*(a*PWM.^3 + b*PWM.^2 + c*PWM + d);

== matlab function PX4_Run_Mode_R2017b/SENSOR_FILTER/SensorData2States/Translational State Estimation/MATLAB Function ==
  data: a_out output; a_in input; Angles input
function a_out  = Correction(a_in, Angles)

b = single([0; 0; 9.81748]);
phi = Angles(1);
theta = Angles(2);
psi = Angles(3);


Rx = [1 0        0;...
      0 cos(phi) -sin(phi);...
      0 sin(phi) cos(phi)];
Ry = [cos(theta) 0 sin(theta);...
      0 1 0;...
      -sin(theta) 0 cos(theta)];
  
Rz = [cos(psi) -sin(psi) 0;...
      sin(psi) cos(psi) 0;...
      0 0 1];
  
% body 2 world rotation
R = Rz * Ry * Rx;  
a_out = R*a_in - b;

== matlab function PX4_Run_Mode_R2017b/RC_FILTER/RC_REF_BIAS ==
  data: RC_IN input; RC_OUT output; CONFIG_CMD input; RESET input; MOV_AVG_WINDOW parameter
function RC_OUT = RCRefBias(RC_IN, CONFIG_CMD, RESET, MOV_AVG_WINDOW)

%% Initiate BIAS memory
persistent BIAS;
if(isempty(BIAS) || RESET)
    BIAS = single([0; 0; 0; 0; 0; 0]);
end

%% If Pre-Armed, average input
if(CONFIG_CMD)
    BIAS = BIAS + RC_IN/MOV_AVG_WINDOW;
end

%% Remove BIAS from input
RC_OUT = RC_IN - BIAS;
RC_OUT(6) = -RC_OUT(6);

== matlab function PX4_Run_Mode_R2017b/SENSOR_FILTER/StateEstimatesInitialConditions/Initial_Filteres_Sensor_Data ==
  data: S output
function S = InitialFilteredSensorData
S = single([0; 0; 0;...             % Magnetometer
            0; 0; 0;...             % Accelerometer
            0; 0; 0;...             % Gyroscope
            0;...                   % Barometer
            0; 0; 0; 0;...          % GPS
            0; 0; 0;...             % Battery
            0]);                    % Sonar

== matlab function PX4_Run_Mode_R2017b/MOTOR_MIXING & MODE_SELECTOR/  ==
  data: Thrust input; Roll input; M1 output; Pitch input; Yaw input; M2 output; M3 output; M4 output; T1 parameter; T2 parameter; T3 parameter; T4 parameter; R1 parameter; R2 parameter; R3 parameter; R4 parameter; P1 parameter; P2 parameter; P3 parameter; P4 parameter; Y1 parameter; Y2 parameter; Y3 parameter; Y4 parameter; PWM_d parameter; PWM_c parameter; PWM_b parameter; PWM_a parameter; type1 output; type2 output
function [M1, M2, M3, M4, type1, type2] = Motor_Mixer(Thrust, Roll, Pitch, Yaw, T1, T2, T3, T4, R1, R2, R3, R4, P1, P2, P3, P4, Y1, Y2, Y3, Y4, PWM_d, PWM_c, PWM_b, PWM_a)

%% New test system
Mm = [T1 T2 T3 T4;...                                       % Thrust in N Motor 1 (Front - Right CCW)
      R1 R2 R3 R4;...                                       % Thrust in N Motor 2 (Rear  - Right  CW)
      P1 P2 P3 P4;...                                       % Thrust in N Motor 3 (Rear  - Left  CCW)
      Y1 Y2 Y3 Y4];                                         % Thrust in N Motor 4 (Front - Left   CW)
M = single([0; 0; 0; 0]);
M = single(inv(Mm)*[-Thrust; Roll; Pitch; Yaw]);
% M(1) = single(T1*Thrust + R1*Roll + P1*Pitch + Y1*Yaw); % Thrust in N Motor 1 (Front - Right CCW)
% M(2) = single(T2*Thrust + R2*Roll + P2*Pitch + Y2*Yaw); % Thrust in N Motor 2 (Rear  - Right  CW)
% M(3) = single(T3*Thrust + R3*Roll + P3*Pitch + Y3*Yaw); % Thrust in N Motor 3 (Rear  - Left  CCW)
% M(4) = single(T4*Thrust + R4*Roll + P4*Pitch + Y4*Yaw); % Thrust in N Motor 4 (Front - Left   CW)

%% NOTES
% Apply correction for battery draining during flight

%% Convert Forces to PWM
a = PWM_a;
b = PWM_b;
c = PWM_c;

type1 = single(0);                % Solver type
type2 = single(0);                % Solver type
sol1 = single([0; 0; 0; 0]);
sol2 = single([0; 0; 0; 0]);
sol3 = single([0; 0; 0; 0]);
fsol = single([0; 0; 0; 0]);

for i = 1:4
    d = PWM_d - M(i);
    r = -1;
    pwm0 = single([(-2*b + sqrt(4*b^2-12*a*c))/(6*a) (-2*b - sqrt(4*b^2-12*a*c))/(6*a)]);

    %% intermediate values defining form of ax^3 + bx^2 + cx + d = 0
    f = ((3*c/a) - (b^2/a^2))/3;
    g = ((2*b^3/a^3) - (9*b*c/a^2) + (27*d/a))/27;
    h = (g^2/4) + (f^3/27);

    if(h>0)
        r = 1;
    elseif(h == 0 && g == 0 && f == 0)
        r = 2;
    elseif(h <= 0)
        r = 3;
    end
    
    %% Switch cases between different solutions
    switch r
        case 1  % only 1 real root
            type1 = type1 + 1*10^(i-1);
            S = nthroot(-(g/2) + sqrt(h),3);
            U = nthroot(-(g/2) - sqrt(h),3);
            sol1(i) = (S+U) - (b/(3*a));                                   % Real Root
            sol2(i) = -(S+U)/2 - (b/(3*a));                                % Real part of imaginary root
            sol3(i) = -(S+U)/2 - (b/(3*a));                                % Real part of imaginary root
            
        case 2  % All three roots are real and equal
            type1 = type1 + 2*10^(i-1);
            sol1(i) = nthroot(-(d/a),3);                                   % Real Root
            sol2(i) = nthroot(-(d/a),3);                                   % Real Root
            sol3(i) = nthroot(-(d/a),3);                                   % Real Root
            
        case 3  % All three roots are real
            type1 = type1 + 3*10^(i-1);
            j = nthroot(sqrt((g^2/4)-h),3);
            k = acos(-g/(2*sqrt((g^2/4)-h)));
            sol1(i) = 2*j*cos(k/3) - (b/(3*a));                            % Real Root
            sol2(i) = -j*(cos(k/3) + sqrt(3)*sin(k/3)) - (b/(3*a));        % Real Root
            sol3(i) = -j*(cos(k/3) - sqrt(3)*sin(k/3)) - (b/(3*a));        % Real Root
    end
            
    %% Find the middle solution
    SOL = [sol1(i); sol2(i); sol3(i)];
    if(sol1(i) >= pwm0(1)-1 && sol1(i) <= pwm0(2)+1)
        fsol(i) = sol1(i);
        type2 = type2 + 1*10^(i-1);
    elseif(sol2(i) >= pwm0(1)-1 && sol2(i) <= pwm0(2)+1)
        fsol(i) = sol2(i);
        type2 = type2 + 2*10^(i-1);
    elseif(sol3(i) >= pwm0(1)-1 && sol3(i) <= pwm0(2)+1)
        fsol(i) = sol3(i);
        type2 = type2 + 3*10^(i-1);
    elseif(M(i) < 3.8)
        fsol(i) = min(SOL);
        type2 = type2 + 4*10^(i-1);
    elseif(M(i) > 3.8)
        fsol(i) = max(SOL);
        type2 = type2 + 5*10^(i-1);
    end
    
    %% Limit the solution between [1000, 2000]
        if(fsol(i) < 1000)
            fsol(i) = 1000;
        elseif(fsol(i) > 2000)
            fsol(i) = 2000;
        end
        
end

%% PWM output
M1 = round(fsol(1));
M2 = round(fsol(2));
M3 = round(fsol(3));
M4 = round(fsol(4));

== matlab function PX4_Run_Mode_R2017b/RC_FILTER/Scale_Yaw_RC ==
  data: RC_Yaw input; RC2_MAX parameter; T_YAW output; RC2_MIN parameter; RC2_TRIM parameter; RC2_DB parameter; YAW_MAX parameter
function T_YAW = Scale_Yaw_RC(RC_Yaw, RC2_MAX, RC2_MIN, RC2_TRIM, RC2_DB, YAW_MAX)

%% Initialize variable
T_YAW = single(0);
RC_Yaw = single(RC_Yaw);

%% Transform RC channel input to desired values
% RC channel 3 [984    , 1499    , 2006]
%              [RC3_MIN, RC3_TRIM, RC3_MAX]

% Test if RC was once connected, or is still connected
T_YAW = RC_Yaw - RC2_TRIM;
if(T_YAW < -RC2_DB)
    T_YAW = T_YAW/(RC2_TRIM - RC2_MIN);
elseif(T_YAW > RC2_DB)
    T_YAW = T_YAW/(RC2_MAX - RC2_TRIM);
else
    T_YAW = single(0);
end


%% Limit output to [-1, 1]
if(RC_Yaw == 0)
    T_YAW = single(0);
else
    if(T_YAW > 1)
        T_YAW = single(1);
    elseif(T_YAW < -1)
        T_YAW = single(-1);
    end
end

%% Scale output to [MIN MAX] Yaw Rate value
T_YAW = T_YAW * YAW_MAX;
if(T_YAW > YAW_MAX)
    T_YAW = single(YAW_MAX);
elseif(T_YAW < -YAW_MAX)
    T_YAW = single(-YAW_MAX);
end

== matlab function PX4_Run_Mode_R2017b/SENSOR_FILTER/Fixed Bias removal and scaling/Gyroscope Calibration/GYRO_BIAS ==
  data: GYRO_IN input; RESET input; CONFIG_CMD input; MOV_AVG_WINDOW parameter; BGYRO output
function BGYRO = GyroBias(GYRO_IN, RESET, CONFIG_CMD, MOV_AVG_WINDOW)

Gx = GYRO_IN(1);
Gy = GYRO_IN(2);
Gz = GYRO_IN(3);

%% Initiate BIAS memory
persistent BIAS;
if(isempty(BIAS) || RESET)
    BIAS = single([0; 0; 0]);
end

BGYRO = single([0; 0; 0]);

%% If Pre-Armed, average input
if(CONFIG_CMD)
    BIAS(1) = BIAS(1) + Gx/MOV_AVG_WINDOW;
    BIAS(2) = BIAS(2) + Gy/MOV_AVG_WINDOW;
    BIAS(3) = BIAS(3) + Gz/MOV_AVG_WINDOW;
end

%% Outputs
BGYRO = BIAS;

== matlab function PX4_Run_Mode_R2017b/RC_FILTER/Scale_Pitch_RC ==
  data: RC_Pitch input; RC3_MAX parameter; T_PITCH output; RC3_MIN parameter; RC3_TRIM parameter; RC3_DB parameter; PITCH_MAX parameter
function T_PITCH = Scale_Pitch_RC(RC_Pitch, RC3_MAX, RC3_MIN, RC3_TRIM, RC3_DB, PITCH_MAX)

%% Initialize variable
T_PITCH = single(0);
RC_Pitch = single(RC_Pitch);

%% Transform RC channel input to desired values
% RC channel 3 [984    , 1499    , 2006]
%              [RC3_MIN, RC3_TRIM, RC3_MAX]

% Test if RC was once connected, or is still connected
T_PITCH = RC_Pitch - RC3_TRIM;
if(T_PITCH < -RC3_DB)
    T_PITCH = T_PITCH/(RC3_TRIM - RC3_MIN);
elseif(T_PITCH > RC3_DB)
    T_PITCH = T_PITCH/(RC3_MAX - RC3_TRIM);
else
    T_PITCH = single(0);
end


%% Limit output to [-1, 1]
if(RC_Pitch == 0)
    T_PITCH = single(0);
else
    if(T_PITCH > 1)
        T_PITCH = single(1);
    elseif(T_PITCH < -1)
        T_PITCH = single(-1);
    end
end

%% Scale output to [MIN MAX] Pitch value
T_PITCH = T_PITCH * PITCH_MAX;
if(T_PITCH > PITCH_MAX)
    T_PITCH = single(PITCH_MAX);
elseif(T_PITCH < -PITCH_MAX)
    T_PITCH = single(-PITCH_MAX);
end

%% Inverse pitch for convenience
T_PITCH = -T_PITCH;

== matlab function PX4_Run_Mode_R2017b/CONTROLLER/Outer Control Loop/Thrust Control/MATLAB Function2 ==
  data: T_z input; Z_Vel_Ref output
function Z_Vel_Ref = Z_Vel_Ref(T_z)

Z_Vel_Ref = (T_z + single(0.5))*single(2);

% if(abs(Z_Vel_Ref) > 0.1)
%     Z_Vel_Ref = sign(Z_Vel_Ref)*single(0.1);
% end

== matlab function PX4_Run_Mode_R2017b/RC_FILTER/Scale_Roll_RC ==
  data: RC_Roll input; T_ROLL output; RC1_MAX parameter; RC1_MIN parameter; RC1_TRIM parameter; RC1_DB parameter; ROLL_MAX parameter
function T_ROLL = Scale_Roll_RC(RC_Roll, RC1_MAX, RC1_MIN, RC1_TRIM, RC1_DB, ROLL_MAX)

%% Initialize variable
T_ROLL = single(0);
RC_Roll = single(RC_Roll);

%% Transform RC channel input to desired values
% RC channel 1 [984    , 1499    , 2006]
%              [RC1_MIN, RC1_TRIM, RC1_MAX]

% Test if RC was once connected, or is still connected
T_ROLL = RC_Roll - RC1_TRIM;
if(T_ROLL < -RC1_DB)
    T_ROLL = T_ROLL/(RC1_TRIM - RC1_MIN);
elseif(T_ROLL > RC1_DB)
    T_ROLL = T_ROLL/(RC1_MAX - RC1_TRIM);
else
    T_ROLL = single(0);
end


%% Limit output to [-1, 1]
if(RC_Roll == 0)
    T_ROLL = single(0);
else
    if(T_ROLL > 1)
        T_ROLL = single(1);
    elseif(T_ROLL < -1)
        T_ROLL = single(-1);
    end
end

%% Scale output to [MIN MAX] Roll value
T_ROLL = T_ROLL * ROLL_MAX;
if(T_ROLL > ROLL_MAX)
    T_ROLL = single(ROLL_MAX);
elseif(T_ROLL < -ROLL_MAX)
    T_ROLL = single(-ROLL_MAX);
end

== matlab function PX4_Run_Mode_R2017b/RC_FILTER/Scale_Throttle_RC1 ==
  data: RC_Thrust input; RC4_MAX parameter; T_Z output; RC4_MIN parameter; RC4_TRIM parameter; RC4_DB parameter; Z_MAX parameter
function T_Z = Scale_Throttle_RC(RC_Thrust, RC4_MAX, RC4_MIN, RC4_TRIM, RC4_DB, Z_MAX)

%% Initialize variable
T_Z = single(0);
RC_Thrust = single(RC_Thrust);

%% Transform RC channel input to desired values
% RC channel 4 [1000    , 1500    , 2000]
%              [RC4_MIN, RC4_TRIM, RC4_MAX]

% Test if RC was once connected, or still is connected
T_Z = RC_Thrust - RC4_TRIM;
if(T_Z < -RC4_DB)
    T_Z = T_Z/(RC4_TRIM - RC4_MIN);
elseif(T_Z > RC4_DB)
    T_Z = T_Z/(RC4_MAX - RC4_TRIM);
else
    T_Z = single(0);
end

%% Limit output to [0, 1]
T_Z = 0.5 * T_Z + 0.5;
if(RC_Thrust == 0)
    T_Z = single(0);
else
    if(T_Z > 1)
        T_Z = single(1);
    elseif(T_Z < 0)
        T_Z = single(0);
    end    
end

%% Scale output to [MIN MAX] Z value
T_Z = T_Z * Z_MAX;
if(T_Z > Z_MAX)
    T_Z = single(Z_MAX);
elseif(T_Z < 0)
    T_Z = single(0);
end

== matlab function PX4_Run_Mode_R2017b/RC_FILTER/Scale_Throttle_RC ==
  data: RC_Throttle input; RC4_MAX parameter; T_THROTTLE output; RC4_MIN parameter
function T_THROTTLE = Scale_Throttle_RC(RC_Throttle, RC4_MAX, RC4_MIN)

%% Initialize variable
T_THROTTLE = single(0);
RC_Throttle = single(RC_Throttle);

%% Limit output to [1000 2000]
if(RC_Throttle ~= single(0))
    if(RC_Throttle > RC4_MAX)
        T_THROTTLE = single(RC4_MAX);
    elseif(RC_Throttle < RC4_MIN)
        T_THROTTLE = single(RC4_MIN);
    else
        T_THROTTLE = RC_Throttle;
    end
else
    T_THROTTLE = single(0);
end

== matlab function PX4_Run_Mode_R2017b/RC_FILTER/Scale_Pitch_RC1 ==
  data: RC_Pitch input; RC3_MAX parameter; T_X output; RC3_MIN parameter; RC3_TRIM parameter; RC3_DB parameter; X_MAX parameter
function T_X = Scale_Pitch_RC(RC_Pitch, RC3_MAX, RC3_MIN, RC3_TRIM, RC3_DB, X_MAX)

%% Initialize variable
T_X = single(0);
RC_Pitch = single(RC_Pitch);

%% Transform RC channel input to desired values
% RC channel 3 [984    , 1499    , 2006]
%              [RC3_MIN, RC3_TRIM, RC3_MAX]

% Test if RC was once connected, or is still connected
T_X = RC_Pitch - RC3_TRIM;
if(T_X < -RC3_DB)
    T_X = T_X/(RC3_TRIM - RC3_MIN);
elseif(T_X > RC3_DB)
    T_X = T_X/(RC3_MAX - RC3_TRIM);
else
    T_X = single(0);
end


%% Limit output to [-1, 1]
if(RC_Pitch == 0)
    T_X = single(0);
else
    if(T_X > 1)
        T_X = single(1);
    elseif(T_X < -1)
        T_X = single(-1);
    end
end

%% Scale output to [MIN MAX] X value
T_X = T_X * X_MAX;
if(T_X > X_MAX)
    T_X = single(X_MAX);
elseif(T_X < -X_MAX)
    T_X = single(-X_MAX);
end

== matlab function PX4_Run_Mode_R2017b/SENSOR_FILTER/Fixed Bias removal and scaling/Accelerometer Calibration/MATLAB Function ==
  data: a input; acor output; CAL_ACC0_XOFFSET parameter; CAL_ACC0_YOFFSET parameter; CAL_ACC0_ZOFFSET parameter; CAL_ACC0_XXSCALE parameter; CAL_ACC0_XYSCALE parameter; CAL_ACC0_XZSCALE parameter; CAL_ACC0_YXSCALE parameter; CAL_ACC0_YYSCALE parameter; CAL_ACC0_YZSCALE parameter; CAL_ACC0_ZXSCALE parameter; CAL_ACC0_ZYSCALE parameter; CAL_ACC0_ZZSCALE parameter
function acor = Accelerometer_Correction(a, CAL_ACC0_XOFFSET, CAL_ACC0_YOFFSET, CAL_ACC0_ZOFFSET, CAL_ACC0_XXSCALE, CAL_ACC0_XYSCALE, CAL_ACC0_XZSCALE, CAL_ACC0_YXSCALE, CAL_ACC0_YYSCALE, CAL_ACC0_YZSCALE, CAL_ACC0_ZXSCALE, CAL_ACC0_ZYSCALE, CAL_ACC0_ZZSCALE)

V = [CAL_ACC0_XOFFSET; CAL_ACC0_YOFFSET; CAL_ACC0_ZOFFSET];      % Bias correction

W = [CAL_ACC0_XXSCALE CAL_ACC0_YXSCALE CAL_ACC0_ZXSCALE;...
     CAL_ACC0_XYSCALE CAL_ACC0_YYSCALE CAL_ACC0_ZYSCALE;...
     CAL_ACC0_XZSCALE CAL_ACC0_YZSCALE CAL_ACC0_ZZSCALE];        % Scaling correction



acor = W*(a - V);

== matlab function PX4_Run_Mode_R2017b/SENSOR_FILTER/Fixed Bias removal and scaling/MagnetoMeter Calibration/MATLAB Function ==
  data: m input; I input; mcor output; CAL_MAG0_XOFFSET parameter; CAL_MAG0_YOFFSET parameter; CAL_MAG0_ZOFFSET parameter; CAL_MAG0_XXSCALE parameter; CAL_MAG0_XYSCALE parameter; CAL_MAG0_XZSCALE parameter; CAL_MAG0_YXSCALE parameter; CAL_MAG0_YYSCALE parameter; CAL_MAG0_YZSCALE parameter; CAL_MAG0_ZXSCALE parameter; CAL_MAG0_ZYSCALE parameter; CAL_MAG0_ZZSCALE parameter; CAL_MAG0_XCURCOR parameter; CAL_MAG0_YCURCOR parameter; CAL_MAG0_ZCURCOR parameter
function mcor = Magnetometer_Correction(m, I, CAL_MAG0_XOFFSET, CAL_MAG0_YOFFSET, CAL_MAG0_ZOFFSET, CAL_MAG0_XXSCALE, CAL_MAG0_XYSCALE, CAL_MAG0_XZSCALE, CAL_MAG0_YXSCALE, CAL_MAG0_YYSCALE, CAL_MAG0_YZSCALE, CAL_MAG0_ZXSCALE, CAL_MAG0_ZYSCALE, CAL_MAG0_ZZSCALE, CAL_MAG0_XCURCOR, CAL_MAG0_YCURCOR, CAL_MAG0_ZCURCOR)

%% Hard Iron Corrections
V = [CAL_MAG0_XOFFSET; CAL_MAG0_YOFFSET; CAL_MAG0_ZOFFSET];      % Bias correction

%% Soft Iron Corrections
W = [CAL_MAG0_XXSCALE CAL_MAG0_YXSCALE CAL_MAG0_ZXSCALE;...
     CAL_MAG0_XYSCALE CAL_MAG0_YYSCALE CAL_MAG0_YZSCALE;...
     CAL_MAG0_XZSCALE CAL_MAG0_YZSCALE CAL_MAG0_ZZSCALE];        % Scaling correction

%% Current corrections
B = [CAL_MAG0_XCURCOR; CAL_MAG0_YCURCOR; CAL_MAG0_ZCURCOR];

%% Output corrected Values
mcor = W*(m - V) - B*I;

== matlab function PX4_Run_Mode_R2017b/SENSOR_FILTER/Fixed Bias removal and scaling/Gyroscope Calibration/MATLAB Function ==
  data: w input; BIAS input; wcor output; CAL_GYRO0_XXSCALE parameter; CAL_GYRO0_XYSCALE parameter; CAL_GYRO0_XZSCALE parameter; CAL_GYRO0_YXSCALE parameter; CAL_GYRO0_YYSCALE parameter; CAL_GYRO0_YZSCALE parameter; CAL_GYRO0_ZXSCALE parameter; CAL_GYRO0_ZYSCALE parameter; CAL_GYRO0_ZZSCALE parameter
function wcor = Gyroscope_Correction(w, BIAS, CAL_GYRO0_XXSCALE, CAL_GYRO0_XYSCALE, CAL_GYRO0_XZSCALE, CAL_GYRO0_YXSCALE, CAL_GYRO0_YYSCALE, CAL_GYRO0_YZSCALE, CAL_GYRO0_ZXSCALE, CAL_GYRO0_ZYSCALE, CAL_GYRO0_ZZSCALE)

V = BIAS;      % Bias correction
W = [CAL_GYRO0_XXSCALE CAL_GYRO0_XYSCALE CAL_GYRO0_XZSCALE;...
     CAL_GYRO0_YXSCALE CAL_GYRO0_YYSCALE CAL_GYRO0_YZSCALE;...
     CAL_GYRO0_ZXSCALE CAL_GYRO0_ZYSCALE CAL_GYRO0_ZZSCALE];        % Scaling correction



wcor = W*(w - V);

== matlab function PX4_Run_Mode_R2017b/SENSOR_FILTER/Fixed Bias removal and scaling/GPS Calibration/MATLAB Function ==
  data: p input; pcor output; CAL_GPS0_YOFFSET parameter; CAL_GPS0_ZOFFSET parameter; CAL_GPS0_XXSCALE parameter; CAL_GPS0_XYSCALE parameter; CAL_GPS0_XZSCALE parameter; CAL_GPS0_YXSCALE parameter; CAL_GPS0_YYSCALE parameter; CAL_GPS0_YZSCALE parameter; CAL_GPS0_ZXSCALE parameter; CAL_GPS0_XOFFSET parameter; CAL_GPS0_ZYSCALE parameter; CAL_GPS0_ZZSCALE parameter; V_IN input
function pcor = GPS_Correction(p, CAL_GPS0_YOFFSET, CAL_GPS0_ZOFFSET, CAL_GPS0_XXSCALE, CAL_GPS0_XYSCALE, CAL_GPS0_XZSCALE, CAL_GPS0_YXSCALE, CAL_GPS0_YYSCALE, CAL_GPS0_YZSCALE, CAL_GPS0_ZXSCALE, CAL_GPS0_XOFFSET, CAL_GPS0_ZYSCALE, CAL_GPS0_ZZSCALE, V_IN)

V = [CAL_GPS0_XOFFSET; CAL_GPS0_YOFFSET; CAL_GPS0_ZOFFSET];      % Bias correction
V = V_IN;

W = [CAL_GPS0_XXSCALE CAL_GPS0_YXSCALE CAL_GPS0_ZXSCALE;...
     CAL_GPS0_XYSCALE CAL_GPS0_YYSCALE CAL_GPS0_ZYSCALE;...
     CAL_GPS0_XZSCALE CAL_GPS0_YZSCALE CAL_GPS0_ZZSCALE];        % Scaling correction



pcor = W*(p - V);

== matlab function PX4_Run_Mode_R2017b/SENSOR_FILTER/Fixed Bias removal and scaling/Battery Calibration/MATLAB Function ==
  data: Bat input; Batcor output; CAL_BAT0_YOFFSET parameter; CAL_BAT0_ZOFFSET parameter; CAL_BAT0_XXSCALE parameter; CAL_BAT0_XYSCALE parameter; CAL_BAT0_XZSCALE parameter; CAL_BAT0_YXSCALE parameter; CAL_BAT0_YYSCALE parameter; CAL_BAT0_YZSCALE parameter; CAL_BAT0_ZXSCALE parameter; CAL_BAT0_XOFFSET parameter; CAL_BAT0_ZYSCALE parameter; CAL_BAT0_ZZSCALE parameter
function Batcor = Battery_Correction(Bat, CAL_BAT0_YOFFSET, CAL_BAT0_ZOFFSET, CAL_BAT0_XXSCALE, CAL_BAT0_XYSCALE, CAL_BAT0_XZSCALE, CAL_BAT0_YXSCALE, CAL_BAT0_YYSCALE, CAL_BAT0_YZSCALE, CAL_BAT0_ZXSCALE, CAL_BAT0_XOFFSET, CAL_BAT0_ZYSCALE, CAL_BAT0_ZZSCALE)

V = [CAL_BAT0_XOFFSET; CAL_BAT0_YOFFSET; CAL_BAT0_ZOFFSET];      % Bias correction
W = [CAL_BAT0_XXSCALE CAL_BAT0_XYSCALE CAL_BAT0_XZSCALE;...
     CAL_BAT0_YXSCALE CAL_BAT0_YYSCALE CAL_BAT0_YZSCALE;...
     CAL_BAT0_ZXSCALE CAL_BAT0_ZYSCALE CAL_BAT0_ZZSCALE];        % Scaling correction



Batcor = inv(W)*(Bat - V);
